simulink model "sampleModel1675"  (R2023a)
settings: Solver=VariableStepAuto  StartTime=0.0  StopTime=10.0  RelTol=1e-3
libraries: hdlsllib x3, simulink x2
settings Model: Creator=user1  LastModifiedBy=user1

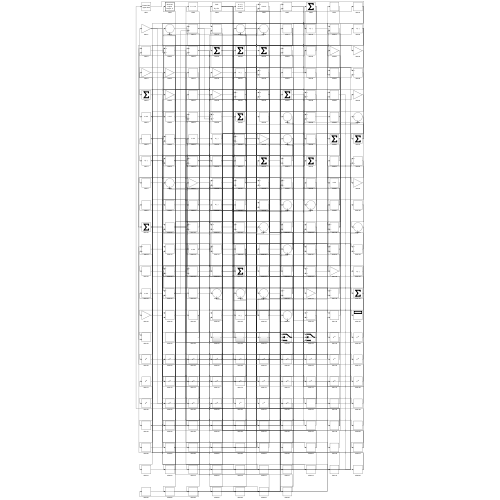
[thumbnail: Simulink's stored preview of the top-level diagram]
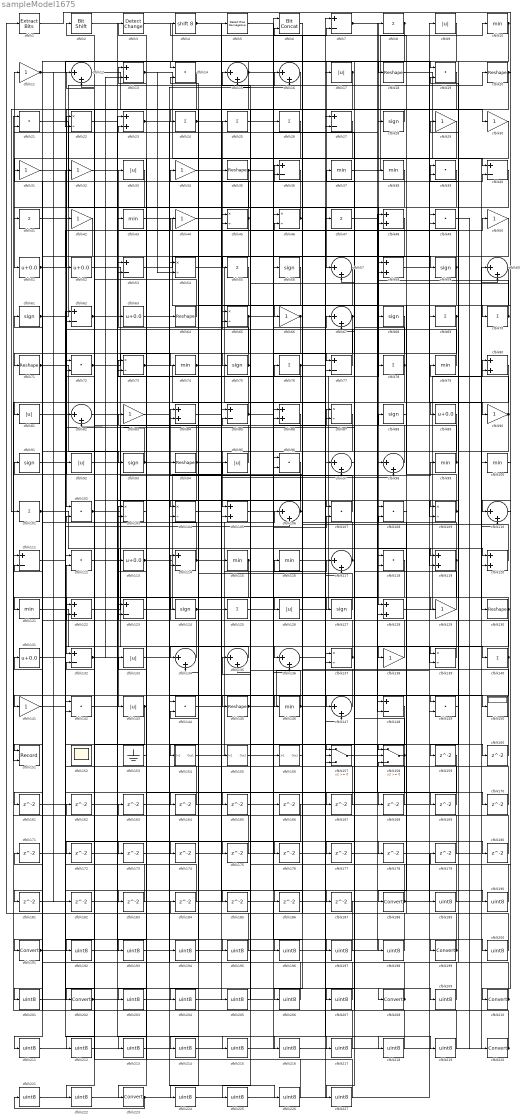
== system sampleModel1675 ==
  cfblk1 : simulink/Logic and Bit Operations/Extract Bits  bitsToExtract=Upper half  numBits=8  bitIdxRange=[0 7]  outScalingMode=Preserve fixed-point scaling
      settings: LibrarySourceBlock=|
      | hdlsllib/Logic and Bit
      | Operations/Extract Bits
  cfblk{10,37..38,43,74,79,99..100,115..116,121,146} (12 alike) : MinMax
  cfblk{8,24..26,41,47,55,69..70,76,78,101,125,140} (14 alike) : Sum  Inputs=+
  cfblk{14,19,21,39,49,72,96,102,107..108,112,118,142,144,149} (15 alike) : DotProduct  OutDataTypeStr=Inherit: Inherit via internal rule
  cfblk{22,45..46,54,65,73,87,103..104,109,137,139} (12 alike) : Product  Inputs=*/  RndMeth=Zero  SaturateOnIntegerOverflow=on
  cfblk{13,23,48,58,80,84,86,105,119..120,122,128} (12 alike) : Sum
  cfblk{12,15..16,57,60,67,82,97..98,106,110,117,134..136,147} (16 alike) : Sum  Inputs=|++
  cfblk{11,29..32,34,42,44,50,66,83,90,129,138,141} (15 alike) : Gain
  cfblk{7,27,36,40,53,62,77,85,111,114,123,132,148} (13 alike) : Sum  Inputs=+-
  cfblk{51..52,63,89,113,131} (6 alike) : Bias  Bias=0.0  SaturateOnIntegerOverflow=off
  cfblk{28,56,59,61,68,75,88,91,93,124,127} (11 alike) : Signum
  cfblk{9,17,33,81,92,95,126,133,143} (9 alike) : Abs  SaturateOnIntegerOverflow=off
  cfblk{18,20,35,64,71,94,130,145} (8 alike) : Reshape
  cfblk150 : Display
  cfblk151 : Record  FileSettingsInternal="{\"entries\":[{\"content\":{\"excelSettings\":{\"content\":{},\"type\":\"Streamout.ExcelSettings\"}},\"type\":\"Streamout.FileSettingStorage\",\"uuid\":\"\"}],\"packageUris\":[\"http:\\/\\/schema.mathworks.com\\/mf0\\/streamout_blocks\\/R2020a\"],\"version\":\"1.0\"}"  Layout=[1 1]  SignalsInternal="{\"entries\":[{\"content\":{\"signals\":[{\"content\":{\"blockPath\":[],\"dimensions\":[1],\"domain\":\"\",\"lineColor\":\"#a2142f\",\"plots\":[1],\"port\":1,\"signalID\":2773,\"signalName\":\"XY Graph:1\"},\"type\":\"RecordBlkView.Signal\",\"uuid\":\"\"},{\"content\":{\"blockPath\":[],\"dimensions\":[1],\"domain\":\"\",\"lineColor\":\"#139fff\",\"plots\":[1],\"port\":2,\"signalID\":2776,\"signalName\":\"XY Graph:2\"},\"type\":\"RecordBlkView.Signal\",\"uuid\":\"\"}]},\"type\":\"RecordBlkView.InputSignals\",\"uuid\":\"\"}],\"packageUris\":[\"http:\\/\\/schema.mathworks.com\\/mf0\\/streamout_blocks\\/R2020a\"],\"version\":\"1.0\"}"  VisualizationBindings="{\"xyplotplugin\":{\"info\":[{\"series\":[{\"bindingParametersList\":[{\"parameter\":\"X-Axis\",\"signalID\":2773,\"signalName\":\"XY Graph:1\"},{\"parameter\":\"Y-Axis\",\"signalID\":2776,\"signalName\":\"XY Graph:2\"}],\"seriesID\":1462}],\"subplotID\":1}]}}"  CompatibilityTag=XY  st=-1
  cfblk152 : Scope
      settings: Floating=on
  cfblk153 : Ground
  cfblk154 : Subsystem
      settings: LibrarySourceBlock=|
      | hdlsllib/Ports &
      | Subsystems/Subsystem
  cfblk155 : Subsystem
      settings: LibrarySourceBlock=|
      | hdlsllib/Ports &
      | Subsystems/Subsystem
  cfblk156 : Subsystem
      settings: LibrarySourceBlock=|
      | hdlsllib/Ports &
      | Subsystems/Subsystem
  cfblk157 : Switch  SaturateOnIntegerOverflow=off  InputSameDT=off
  cfblk158 : Switch  SaturateOnIntegerOverflow=off  InputSameDT=off
  cfblk{159..187} (29 alike) : Delay  SampleTime=1
  cfblk{188,191,199,202,208,210,220,223} (8 alike) : DataTypeConversion  SaturateOnIntegerOverflow=off  RndMeth=Floor
  cfblk{189..190,192..198,200..201,203..207,209,211..219,221..222,224..227} (32 alike) : DataTypeConversion  OutDataTypeStr=uint8  SaturateOnIntegerOverflow=off  RndMeth=Floor
  cfblk2 : hdlsllib/Logic and Bit Operations/Bit Shift  mode=Shift Left Logical  N=0
  cfblk3 : simulink/Logic and Bit Operations/Detect Change  vinit=0  OutDataTypeStr=boolean
      settings: LibrarySourceBlock=|
      | hdlsllib/Logic and Bit
      | Operations/Detect
      | Change
  cfblk4 : ArithShift  BitShiftNumber=8
  cfblk5 : hdlsllib/Logic and Bit Operations/Detect Rise Nonnegative  vinit=0  OutDataTypeStr=boolean
  cfblk6 : hdlsllib/Logic and Bit Operations/Bit Concat  numInputs=2
  wires:
  cfblk72/1 -> cfblk74/1, cfblk209/1
  cfblk128/1 -> cfblk80/1
  cfblk67/1 -> cfblk71/1, cfblk177/1
  cfblk16/1 -> cfblk101/1
  cfblk3/1 -> cfblk57/1
  cfblk143/1 -> cfblk13/1, cfblk172/1
  cfblk126/1 -> cfblk8/1
  cfblk96/1 -> cfblk202/1
  cfblk87/1 -> cfblk105/1
  cfblk77/1 -> cfblk25/1
  cfblk107/1 -> cfblk84/1
  cfblk61/1 -> cfblk16/1, cfblk158/2
  cfblk112/1 -> cfblk120/1
  cfblk18/1 -> cfblk40/1
  cfblk154/1(Out1) -> cfblk117/1
  cfblk45/1 -> cfblk11/1, cfblk104/2
  cfblk117/1 -> cfblk94/1, cfblk73/1
  cfblk53/1 -> cfblk59/1
  cfblk74/1 -> cfblk98/2, cfblk200/1
  cfblk94/1 -> cfblk147/1, cfblk119/2, cfblk72/1, cfblk192/1
  cfblk114/1 -> cfblk61/1, cfblk148/2
  cfblk64/1 -> cfblk2/1
  cfblk127/1 -> cfblk34/1
  cfblk17/1 -> cfblk102/1, cfblk65/2, cfblk104/1
  cfblk85/1 -> cfblk56/1, cfblk28/1, cfblk73/2
  cfblk57/1 -> cfblk154/1(In1)
  cfblk1/1 -> cfblk70/1
  cfblk113/1 -> cfblk106/1, cfblk63/1
  cfblk13/1 -> cfblk130/1, cfblk54/2
  cfblk101/1 -> cfblk143/1, cfblk140/1
  cfblk98/1 -> cfblk15/1
  cfblk106/1 -> cfblk22/1, cfblk36/1
  cfblk66/1 -> cfblk121/1, cfblk72/2
  cfblk102/1 -> cfblk99/1, cfblk78/1, cfblk190/1
  cfblk122/1 -> cfblk85/2
  cfblk99/1 -> cfblk37/1, cfblk88/1
  cfblk46/1 -> cfblk42/1, cfblk146/1
  cfblk75/1 -> cfblk33/1, cfblk225/1
  cfblk21/1 -> cfblk128/1
  cfblk33/1 -> cfblk81/1
  cfblk105/1 -> cfblk157/1
  cfblk28/1 -> cfblk24/1
  cfblk132/1 -> cfblk13/2, cfblk160/1
  cfblk123/1 -> cfblk45/1
  cfblk12/1 -> cfblk69/1
  cfblk104/1 -> cfblk20/1
  cfblk149/1 -> cfblk79/1
  cfblk118/1 -> cfblk132/1
  cfblk58/1 -> cfblk90/1
  cfblk93/1 -> cfblk64/1, cfblk82/2
  cfblk42/1 -> cfblk151/1
  cfblk62/1 -> cfblk136/1, cfblk216/1
  cfblk116/1 -> cfblk47/1
  cfblk121/1 -> cfblk156/1(In1)
  cfblk23/1 -> cfblk149/1, cfblk128/2
  cfblk51/1 -> cfblk50/1, cfblk197/1
  cfblk100/1 -> cfblk210/1
  cfblk30/1 -> cfblk109/1
  cfblk78/1 -> cfblk151/2, cfblk46/2
  cfblk124/1 -> cfblk87/1, cfblk125/1
  cfblk95/1 -> cfblk3/1
  cfblk19/1 -> cfblk135/2
  cfblk63/1 -> cfblk16/2
  cfblk90/1 -> cfblk129/1, cfblk29/1
  cfblk37/1 -> cfblk10/1
  cfblk145/1 -> cfblk9/1, cfblk187/1
  cfblk11/1 -> cfblk30/1, cfblk18/1, cfblk182/1
  cfblk158/1 -> cfblk82/1, cfblk164/1
  cfblk108/1 -> cfblk188/1
  cfblk7/1 -> cfblk38/1, cfblk150/1
  cfblk26/1 -> cfblk51/1
  cfblk139/1 -> cfblk114/1
  cfblk52/1 -> cfblk124/1
  cfblk27/1 -> cfblk223/1
  cfblk54/1 -> cfblk97/1
  cfblk50/1 -> cfblk66/1
  cfblk138/1 -> cfblk103/1
  cfblk38/1 -> cfblk75/1
  cfblk135/1 -> cfblk134/1
  cfblk140/1 -> cfblk31/1, cfblk141/1
  cfblk24/1 -> cfblk120/2, cfblk119/1
  cfblk20/1 -> cfblk105/2, cfblk41/1, cfblk110/1
  cfblk130/1 -> cfblk126/1, cfblk158/1
  cfblk137/1 -> cfblk95/1, cfblk116/1
  cfblk10/1 -> cfblk22/2, cfblk159/1
  cfblk29/1 -> cfblk145/1
  cfblk129/1 -> cfblk23/2
  cfblk125/1 -> cfblk67/1
  cfblk69/1 -> cfblk89/1, cfblk134/2
  cfblk134/1 -> cfblk112/2
  cfblk141/1 -> cfblk106/2
  cfblk109/1 -> cfblk39/1, cfblk4/1
  cfblk36/1 -> cfblk55/1
  cfblk44/1 -> cfblk5/1
  cfblk5/1 -> cfblk77/1
  cfblk153/1 -> cfblk113/1
  cfblk86/1 -> cfblk191/1
  cfblk43/1 -> cfblk98/1
  cfblk47/1 -> cfblk68/1
  cfblk14/1 -> cfblk52/1
  cfblk115/1 -> cfblk201/1, cfblk213/1
  cfblk142/1 -> cfblk199/1
  cfblk34/1 -> cfblk115/1
  cfblk35/1 -> cfblk92/1, cfblk7/2
  cfblk59/1 -> cfblk118/1, cfblk44/1
  cfblk120/1 -> cfblk76/1
  cfblk88/1 -> cfblk138/1
  cfblk8/1 -> cfblk127/1, cfblk161/1
  cfblk131/1 -> cfblk208/1
  cfblk9/1 -> cfblk39/2
  cfblk71/1 -> cfblk93/1, cfblk176/1
  cfblk79/1 -> cfblk62/2
  cfblk48/1 -> cfblk122/1
  cfblk40/1 -> cfblk77/2
  cfblk49/1 -> cfblk220/1
  cfblk73/1 -> cfblk155/1(In1), cfblk40/2
  cfblk103/1 -> cfblk53/1
  cfblk119/1 -> cfblk43/1, cfblk227/1
  cfblk32/1 -> cfblk109/2
  cfblk84/1 -> cfblk118/2
  cfblk15/1 -> cfblk14/1, cfblk53/2, cfblk19/1, cfblk178/1
  cfblk147/1 -> cfblk21/2
  cfblk76/1 -> cfblk157/2, cfblk224/1
  cfblk4/1 -> cfblk157/3, cfblk36/2, cfblk139/2, cfblk97/2
  cfblk65/1 -> cfblk139/1, cfblk123/2, cfblk180/1
  cfblk22/1 -> cfblk107/1
  cfblk155/1(Out1) -> cfblk107/2
  cfblk2/1 -> cfblk114/2
  cfblk146/1 -> cfblk91/1, cfblk147/2
  cfblk70/1 -> cfblk58/2, cfblk45/2
  cfblk160/1 -> cfblk84/2
  cfblk161/1 -> cfblk149/2
  cfblk162/1 -> cfblk48/1
  cfblk163/1 -> cfblk137/2
  cfblk164/1 -> cfblk132/2
  cfblk82/1 -> cfblk165/1
  cfblk165/1 -> cfblk117/2
  cfblk97/1 -> cfblk167/1
  cfblk167/1 -> cfblk54/1
  cfblk25/1 -> cfblk168/1
  cfblk168/1 -> cfblk85/1
  cfblk91/1 -> cfblk169/1
  cfblk169/1 -> cfblk23/1
  cfblk157/1 -> cfblk170/1
  cfblk170/1 -> cfblk112/1
  cfblk171/1 -> cfblk80/2
  cfblk172/1 -> cfblk136/2
  cfblk31/1 -> cfblk173/1
  cfblk55/1 -> cfblk174/1
  cfblk174/1 -> cfblk46/1
  cfblk148/1 -> cfblk175/1
  cfblk175/1 -> cfblk21/1
  cfblk110/1 -> cfblk179/1
  cfblk179/1 -> cfblk57/2
  cfblk180/1 -> cfblk122/2
  cfblk39/1 -> cfblk181/1
  cfblk181/1 -> cfblk65/1
  cfblk182/1 -> cfblk123/1
  cfblk81/1 -> cfblk183/1
  cfblk183/1 -> cfblk12/2
  cfblk184/1 -> cfblk62/1
  cfblk68/1 -> cfblk185/1
  cfblk156/1(Out1) -> cfblk186/1
  cfblk186/1 -> cfblk58/1
  cfblk187/1 -> cfblk1/1
  cfblk188/1 -> cfblk110/2, cfblk148/1, cfblk15/2
  cfblk178/1 -> cfblk189/1
  cfblk189/1 -> cfblk108/1
  cfblk190/1 -> cfblk108/2
  cfblk191/1 -> cfblk103/2, cfblk17/1
  cfblk192/1 -> cfblk86/1
  cfblk159/1 -> cfblk193/1
  cfblk193/1 -> cfblk86/2
  cfblk83/1 -> cfblk194/1
  cfblk194/1 -> cfblk48/2
  cfblk92/1 -> cfblk195/1
  cfblk195/1 -> cfblk83/1
  cfblk6/1 -> cfblk196/1
  cfblk196/1 -> cfblk137/1
  cfblk197/1 -> cfblk6/1
  cfblk185/1 -> cfblk198/1
  cfblk198/1 -> cfblk6/2
  cfblk199/1 -> cfblk163/1, cfblk162/1, cfblk158/3
  cfblk200/1 -> cfblk142/1
  cfblk201/1 -> cfblk142/2
  cfblk202/1 -> cfblk26/1, cfblk222/1
  cfblk173/1 -> cfblk203/1
  cfblk203/1 -> cfblk96/1
  cfblk56/1 -> cfblk204/1
  cfblk204/1 -> cfblk96/2
  cfblk144/1 -> cfblk205/1
  cfblk205/1 -> cfblk35/1
  cfblk89/1 -> cfblk206/1
  cfblk206/1 -> cfblk144/1
  cfblk177/1 -> cfblk207/1
  cfblk207/1 -> cfblk144/2
  cfblk208/1 -> cfblk184/1, cfblk14/2
  cfblk209/1 -> cfblk131/1
  cfblk210/1 -> cfblk19/2, cfblk135/1
  cfblk80/1 -> cfblk211/1
  cfblk211/1 -> cfblk100/1
  cfblk166/1 -> cfblk212/1
  cfblk212/1 -> cfblk102/2
  cfblk213/1 -> cfblk166/1
  cfblk60/1 -> cfblk214/1
  cfblk214/1 -> cfblk7/1
  cfblk41/1 -> cfblk215/1
  cfblk215/1 -> cfblk60/1
  cfblk216/1 -> cfblk60/2
  cfblk111/1 -> cfblk217/1
  cfblk217/1 -> cfblk12/1
  cfblk136/1 -> cfblk218/1
  cfblk218/1 -> cfblk111/1
  cfblk176/1 -> cfblk219/1
  cfblk219/1 -> cfblk111/2
  cfblk220/1 -> cfblk171/1, cfblk67/2
  cfblk221/1 -> cfblk49/1
  cfblk222/1 -> cfblk49/2
  cfblk223/1 -> cfblk221/1, cfblk87/2
  cfblk224/1 -> cfblk27/1
  cfblk225/1 -> cfblk27/2
  cfblk133/1 -> cfblk226/1
  cfblk226/1 -> cfblk32/1
  cfblk227/1 -> cfblk133/1

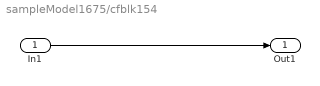
== system sampleModel1675/cfblk154 ==
  In1 : Inport
  Out1 : Outport
  wires:
  In1/1 -> Out1/1

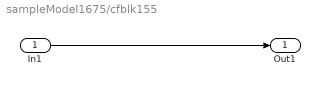
== system sampleModel1675/cfblk155 ==
  In1 : Inport
  Out1 : Outport
  wires:
  In1/1 -> Out1/1

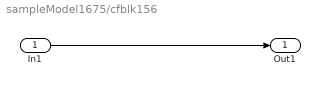
== system sampleModel1675/cfblk156 ==
  In1 : Inport
  Out1 : Outport
  wires:
  In1/1 -> Out1/1
